simulink model "Que_5"  (R2020b)
settings: Solver=VariableStepAuto  StartTime=0.0  StopTime=10.0  RelTol=1e-3
model workspace (MAT data in the model file):
  C = 1e-06
  K1 = 1000000
  K2 = 10
  R = 10
settings Model: Creator=hp  LastModifiedBy=hp

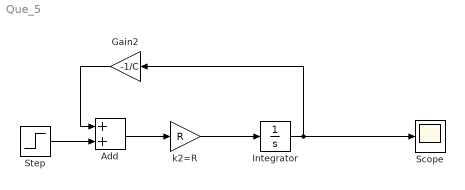
== system Que_5 ==
  Add : Sum
  Gain2 : Gain  Gain=-1/C
  Integrator : Integrator
  Scope : Scope
  Step : Step  SampleTime=0.1
  k2=R : Gain  Gain=R
  wires:
  Gain2/1 -> Add/1
  k2=R/1 -> Integrator/1
  Add/1 -> k2=R/1
  Step/1 -> Add/2
  Integrator/1 -> Scope/1, Gain2/1
